simulink model "Cruise_Control"  (R2018b)
settings: Solver=VariableStepAuto  StartTime=0.0  StopTime=100  RelTol=1e-3
settings Model: Creator=carlos  LastModifiedBy=carlos

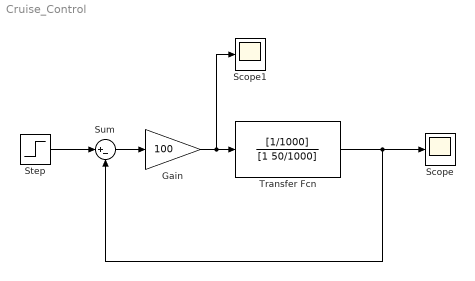
== system Cruise_Control ==
  Gain : Gain  Gain=100
  Scope : Scope
  Scope1 : Scope
  Step : Step  Time=0  After=65  SampleTime=0
  Sum : Sum  Inputs=|+-
  Transfer Fcn : TransferFcn  Numerator=[1/1000]  Denominator=[1 50/1000]
  wires:
  Transfer Fcn/1 -> Sum/2, Scope/1
  Step/1 -> Sum/1
  Gain/1 -> Scope1/1, Transfer Fcn/1
  Sum/1 -> Gain/1
